simulink model "sim_IMP"  (R2018a)
settings: Solver=ode1  StartTime=0.0  StopTime=20  FixedStep=0.002  RelTol=1e-3  EnableMultiTasking=on
values from neighbouring files (symbols this model uses):
  A = [0 1; 0 -1]    [IMP_LQR_Design_Seperation.m]
  A_aug = [A B*Cref; zeros(2,2) Aref]    [IMP_LQR_Design_Seperation.m]
  B = [0 ;2]    [IMP_LQR_Design_Seperation.m]
  B_aug = [B; zeros(2,1)]    [IMP_LQR_Design_Seperation.m]
  C = [1 0]    [IMP_LQR_Design_Seperation.m]
  C_aug = [C zeros(1,2)]    [IMP_LQR_Design_Seperation.m]
  J = J'    [IMP_LQR_Design_Seperation.m]
  K = [K Cref]    [IMP_LQR_Design_Seperation.m]
  N = C_aug*K'    [IMP_LQR_Design_Seperation.m]
  w1 = 2*pi()/5    [IMP_LQR_Design_Seperation.m]
settings Model: ExtModeTrigDuration=5000  Creator=MLevis  LastModifiedBy=jakelangton
settings SolverCC: PositivePriorityOrder=on
settings DataIOCC: LimitDataPoints=on  SaveFormat=Array
settings OptimizationCC: LifeSpan=inf
settings DebuggingCC: SolverPrmCheckMsg=warning  SFUnexpectedBacktrackingDiag=warning  SFNoUnconditionalDefaultTransitionDiag=warning  SFExecutionAtInitializationDiag=none
settings HardwareCC: ProdBitPerPointer=32  ProdBitPerSizeT=32  ProdBitPerPtrDiffT=32  ProdLargestAtomicFloat=None  ProdIntDivRoundTo=Undefined  ProdEndianess=Unspecified  ProdWordSize=32  ProdHWDeviceType=32-bit Generic
settings ModelReferenceCC: PropagateSignalLabelsOutOfModel=off
settings RTWCC: SystemTargetFile=quarc_win64.tlc  TemplateMakefile=quarc_default_tmf  Description=QUARC Win64 Target
settings CodeAppCC: StateflowObjectComments=on
settings STFCustomTargetCC: TargetPreCompLibLocation=C:\PROGRA~3\QUARC\lib\2014a\win64\release  ConcurrentExecutionCompliant=on  GeneratePreprocessorConditionals=Disable all  SystemTargetFile=quarc_win64.tlc
settings GRTTargetCC: TargetPreCompLibLocation=C:\PROGRA~3\QUARC\lib\2014a\win64\release  TargetLangStandard=C89/C90 (ANSI)  ParMdlRefBuildCompliant=off  CompOptLevelCompliant=off  GeneratePreprocessorConditionals=Disable all  CombineOutputUpdateFcns=off  MatFileLogging=off  CPPClassGenCompliant=off  GRTInterface=on  UseToolchainInfoCompliant=off  ExtMode=on  ExtModeMexFile=quarc_comm
settings ConfigComp: CovMetricSettings=dw  CovHtmlReporting=on  CovSaveCumulativeToWorkspaceVar=on  CovSaveSingleToWorkspaceVar=on  CovExternalEMLEnable=off  CovSFcnEnable=off

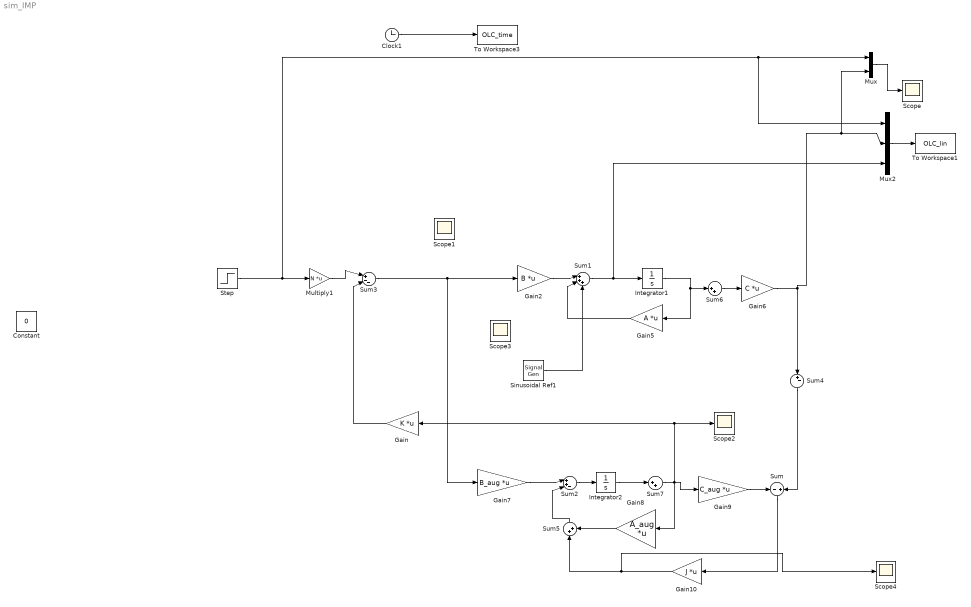
== system sim_IMP ==
  Clock1 : Clock
  Constant : Constant  Value=0
  Gain : Gain  Gain=K  Multiplication=Matrix(K*u)
  Gain10 : Gain  Gain=J  Multiplication=Matrix(K*u)
  Gain2 : Gain  Gain=B  Multiplication=Matrix(K*u)
  Gain5 : Gain  Gain=A  Multiplication=Matrix(K*u)
  Gain6 : Gain  Gain=C  Multiplication=Matrix(K*u)
  Gain7 : Gain  Gain=B_aug  Multiplication=Matrix(K*u)
  Gain8 : Gain  Gain=A_aug  Multiplication=Matrix(K*u)
  Gain9 : Gain  Gain=C_aug  Multiplication=Matrix(K*u)
  Integrator1 : Integrator
  Integrator2 : Integrator
  Multiply1 : Gain  Gain=N  Multiplication=Matrix(K*u)
  Mux : Mux  Inputs=2
  Mux2 : Mux  Inputs=3
  Scope{,1..4} (5 alike) : Scope
  Sinusoidal Ref1 : SignalGenerator  Amplitude=0.5  Frequency=w1  Units=rad/sec
  Step : Step  SampleTime=0
  Sum : Sum  Inputs=-+
  Sum1 : Sum  Inputs=|+++
  Sum2 : Sum  Inputs=|++-
  Sum3 : Sum  Inputs=|+--
  Sum4 : Sum  Inputs=|+-
  Sum5 : Sum  Inputs=|++
  Sum6 : Sum  Inputs=|++
  Sum7 : Sum  Inputs=|++
  To Workspace1 : ToWorkspace  VariableName=OLC_lin  SampleTime=-1
  To Workspace3 : ToWorkspace  VariableName=OLC_time  SampleTime=-1
  wires:
  Clock1/1 -> To Workspace3/1
  Mux2/1 -> To Workspace1/1
  Integrator1/1 -> Sum6/1, Gain5/1
  Gain5/1 -> Sum1/2
  Gain6/1 -> Mux/2, Mux2/2, Sum4/1
  Gain2/1 -> Sum1/1
  Sum1/1 -> Mux2/3, Integrator1/1
  Sum7/1 -> Gain8/1, Scope2/1, Gain/1, Gain9/1
  Sum5/1 -> Sum2/2
  Gain8/1 -> Sum5/2
  Gain9/1 -> Sum/1
  Gain10/1 -> Scope4/1, Sum5/1
  Sum/1 -> Gain10/1
  Gain7/1 -> Sum2/1
  Mux/1 -> Scope/1
  Sum4/1 -> Sum/2
  Sum6/1 -> Gain6/1
  Sinusoidal Ref1/1 -> Sum1/3
  Integrator2/1 -> Sum7/1
  Sum3/1 -> Gain7/1, Gain2/1
  Step/1 -> Mux2/1, Mux/1, Multiply1/1
  Sum2/1 -> Integrator2/1
  Multiply1/1 -> Sum3/1
  Gain/1 -> Sum3/2
